simulink model "sim660"  (R2025a)
settings: Solver=ode23s  StartTime=0.0  StopTime=10000  RelTol=1e-3
model workspace (MAT data in the model file):
  op_snapshot1 : opcond.OperatingPoint (value not decoded)
undefined symbols (not defined in the file or in its folder): State132MW, State198MW, State198MW_DELAY
libraries: slpidlib x4, simulink x2, adrc_toolbox_library x1
(part 3 of 5)

== matlab function sim660/Subsystem/MATLAB Function1 ==
  data: NE input; hst input; dNE output; hfw input; Dst input; eta input
function dNE= dNE(NE,hst,hfw,Dst,eta)
%#codegen
Ttb=10;

%eta=330e3/(3610.61-1058.93)/224.09;%0.5771188421
%eta=264e3/(3625.6-1014.34)/198.243;%0.5099832937
%eta=198e3/(3630.43-943.45)/160.617;%0.4587850384
%eta=132e3/(3535.09-900)/112.98;%0.4433808
dNE= (-NE+eta*(hst-hfw)*Dst)/Ttb;
end
